simulink model "TxArray_2layers"  (R2021b)
settings: Solver=FixedStepDiscrete  StartTime=0.0  StopTime=100  FixedStep=1e-2  RelTol=1e-3  EnableMultiTasking=on
libraries: raspberrypiNetworklib x8, realtime_pacer_lib x1
settings Model: PacingRate=1000  Creator=Blade  LastModifiedBy=Blade
settings SolverCC: PositivePriorityOrder=on

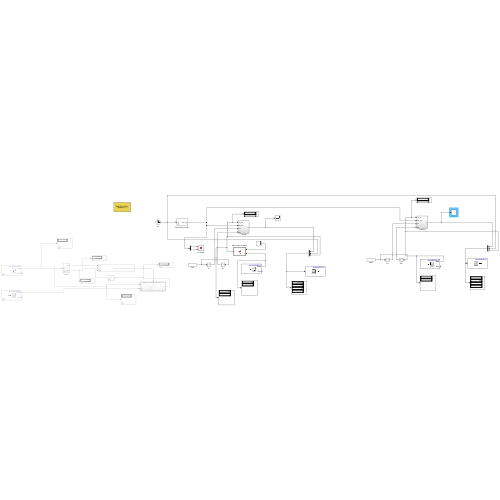
[thumbnail: Simulink's stored preview of the top-level diagram]
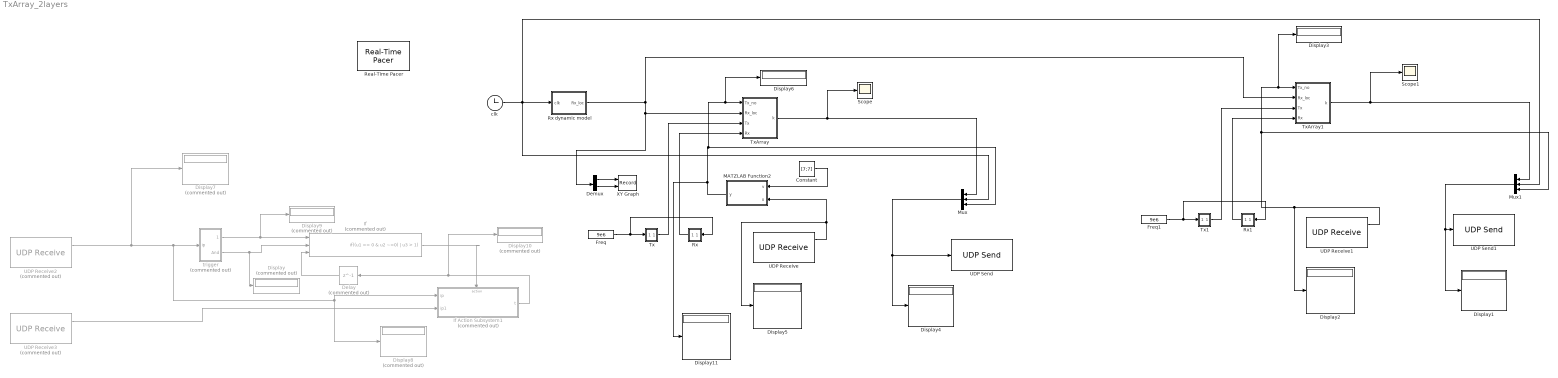
== system TxArray_2layers ==
  Constant : Constant  Value=[7;7]  VectorParams1D=off
  Delay : Delay  Commented=on  DelayLength=1  InitialCondition=0
  Demux : Demux  Outputs=2
  Display{,7..10} (5 alike) : Display  Commented=on
  Display{1..6,11} (7 alike) : Display
  Freq : Constant  Value=9e6
  Freq1 : Constant  Value=9e6
  If : If  Commented=on  NumInputs=3  IfExpression=(u1 == 0 & u2 ~=0) | u3 > 1  ShowElse=off
  If Action Subsystem1 : Subsystem  Commented=on  TreatAsAtomicUnit=on
  MATZLAB Function2 : MATLAB Function  TreatAsAtomicUnit=on
  Mux : Mux  Inputs=3
  Mux1 : Mux  Inputs=3
  Real-Time Pacer : realtime_pacer_lib/Real-Time Pacer  simTimePerRealTime=1
      settings: SourceProductName=Real-Time Pacer
  Rx : Subsystem  mask{dout=1/3*100e-3, phi=0.15, s=800e-6, w=1200e-6, CP=0, SR=0.01}
      mask prompts: dout "out diameter"; phi "fillfact"; s "track spacing"; w "track width"; CP "parasitic capacitance"; SR "source resistance"
      mask TypeOptions dout: Constant1/Value
      mask TypeOptions phi: Constant2/Value
      mask TypeOptions s: Constant3/Value
      mask TypeOptions w: Constant4/Value
      mask TypeOptions CP: Constant6/Value
      mask TypeOptions SR: Constant7/Value
  "Rx dynamic model " : Subsystem  mask{initx=1/2*100e-3*(7+1), inity=1/2*100e-3*(7+1), v_min=[0.01,0.01], v_max=[0.01,0.01]}
      mask prompts: initx "Rx initial x"; inity "Rx initial y"; v_min "Rx min speed"; v_max "Rx max speed"
      mask TypeOptions initx: Delay1/InitialCondition
      mask TypeOptions inity: Delay2/InitialCondition
      mask TypeOptions v_min: Constant/Value
      mask TypeOptions v_max: Constant1/Value
  Rx1 : Subsystem  mask{dout=1/3*100e-3, phi=0.15, s=800e-6, w=1200e-6, CP=0, SR=0.01}
      mask prompts: dout "out diameter"; phi "fillfact"; s "track spacing"; w "track width"; CP "parasitic capacitance"; SR "source resistance"
      mask TypeOptions dout: Constant1/Value
      mask TypeOptions phi: Constant2/Value
      mask TypeOptions s: Constant3/Value
      mask TypeOptions w: Constant4/Value
      mask TypeOptions CP: Constant6/Value
      mask TypeOptions SR: Constant7/Value
  Scope : Scope
  Scope1 : Scope
  Tx : Subsystem  mask{dout=100e-3, phi=0.25, s=3*2500e-6, w=2500e-6, CP=0, SR=0.01}
      mask prompts: dout "out diameter"; phi "fillfact"; s "track spacing"; w "track width"; CP "parasitic capacitance"; SR "source resistance"
      mask TypeOptions dout: Constant1/Value
      mask TypeOptions phi: Constant2/Value
      mask TypeOptions s: Constant3/Value
      mask TypeOptions w: Constant4/Value
      mask TypeOptions CP: Constant6/Value
      mask TypeOptions SR: Constant7/Value
  Tx1 : Subsystem  mask{dout=100e-3, phi=0.25, s=3*2500e-6, w=2500e-6, CP=0, SR=0.01}
      mask prompts: dout "out diameter"; phi "fillfact"; s "track spacing"; w "track width"; CP "parasitic capacitance"; SR "source resistance"
      mask TypeOptions dout: Constant1/Value
      mask TypeOptions phi: Constant2/Value
      mask TypeOptions s: Constant3/Value
      mask TypeOptions w: Constant4/Value
      mask TypeOptions CP: Constant6/Value
      mask TypeOptions SR: Constant7/Value
  TxArray : Subsystem
  TxArray1 : Subsystem
  UDP Receive : raspberrypiNetworklib/UDP Receive  localURL='0.0.0.0'  localPort=2000  remoteURL='0.0.0.0'  remotePort=-1  recvBufferSize=8192  signalDatatype=double  dims=2  isVarSize=off  showBlockingTime=off  blockingTime=0  sampletime=-1  blockPlatform=Raspberry Pi
      settings: SourceProductBaseCode=RASPPI
  UDP Receive1 : raspberrypiNetworklib/UDP Receive  localURL='0.0.0.0'  localPort=2100  remoteURL='0.0.0.0'  remotePort=-1  recvBufferSize=8192  signalDatatype=double  dims=2  isVarSize=off  showBlockingTime=off  blockingTime=0  sampletime=-1  blockPlatform=Raspberry Pi
      settings: SourceProductBaseCode=RASPPI
  UDP Receive2 : raspberrypiNetworklib/UDP Receive  Commented=on  localURL='0.0.0.0'  localPort=1000  remoteURL='0.0.0.0'  remotePort=-1  recvBufferSize=8192  signalDatatype=double  dims=4  isVarSize=off  showBlockingTime=off  blockingTime=0  sampletime=-1  blockPlatform=Raspberry Pi
      settings: SourceProductBaseCode=RASPPI
  UDP Receive3 : raspberrypiNetworklib/UDP Receive  Commented=on  localURL='0.0.0.0'  localPort=1100  remoteURL='0.0.0.0'  remotePort=-1  recvBufferSize=8192  signalDatatype=double  dims=4  isVarSize=off  showBlockingTime=off  blockingTime=0  sampletime=-1  blockPlatform=Raspberry Pi
      settings: SourceProductBaseCode=RASPPI
  UDP Send : raspberrypiNetworklib/UDP Send  remoteURL='172.20.10.3'  remotePort=1000  localURL='0.0.0.0'  localPortSource=Automatically determine  localPort=-1  sampletime=-1  blockPlatform=Raspberry Pi  separateLengthPort=0
      settings: SourceProductBaseCode=RASPPI
  UDP Send1 : raspberrypiNetworklib/UDP Send  remoteURL='172.20.10.3'  remotePort=1100  localURL='0.0.0.0'  localPortSource=Automatically determine  localPort=-1  sampletime=-1  blockPlatform=Raspberry Pi  separateLengthPort=0
      settings: SourceProductBaseCode=RASPPI
  XY Graph : Record  RecordToWorkspace=on  FileSettingsInternal="{\"entries\":[{\"content\":{\"excelSettings\":{\"content\":{},\"type\":\"Streamout.ExcelSettings\"}},\"type\":\"Streamout.FileSettingStorage\",\"uuid\":\"7534ccee-690c-42fe-b6df-7a669e2e1ce8\"}],\"packageUris\":[\"http://schema.mathworks.com/mf0/streamout_blocks/R2020a\"],\"version\":\"1.0\"}"  Layout=[1 1]  SignalsInternal="{\"entries\":[{\"content\":{\"signals\":[{\"content\":{\"blockPath\":[\"TxArray_2layers/XY Graph\"],\"channel\":[],\"dimensions\":[1],\"domain\":\"TxArray_2layers/XY Graph\",\"lineColor\":\"#a2142f\",\"plots\":[1],\"port\":1,\"sid\":[\"\"],\"signalID\":68672,\"signalName\":\"Demux:1\"},\"type\":\"RecordBlkView.Signal\",\"uuid\":\"5f268e60-035f-43e2-bfa9-f0f9b2fdeea8\"},{\"content\":{\"blockPath\":[\"TxArray_2layers/XY Graph\"],\"channel\":[],\"dimensions\":[1],\"domain\":\"TxArray_2layers/XY Graph\",\"lineColor\":\"#139fff\",\"plots\":[1],\"port\":2,\"sid\":[\"\"],\"signalID\":68676,\"signalName\":\"Demux:2\"},\"type\":\"RecordBlkView.Signal\",\"uuid\":\"7309d32f-aeee-4568-9c87-cfd759c20a08\"}]},\"type\":\"RecordBlkView.InputSignals\",\"uuid\":\"395885cf-4d5c-428c-bf2f-d29e5771728a\"}],\"packageUris\":[\"http://schema.mathworks.com/mf0/streamout_blocks/R2020a\"],\"version\":\"1.0\"}"  VisualizationBindings="{\"xyplotplugin\":{\"info\":[{\"series\":[{\"bindingParametersList\":[{\"parameter\":\"X-Axis\",\"signalID\":68672,\"signalName\":\"Demux:1\"},{\"parameter\":\"Y-Axis\",\"signalID\":68676,\"signalName\":\"Demux:2\"}],\"seriesID\":52649}],\"subplotID\":1}]}}"  CompatibilityTag=XY
  clk : Clock
  trigger : Subsystem  Commented=on
  wires:
  Mux1/1 -> Display1/1, UDP Send1/1
  Freq1/1 -> Rx1/1(In1), Tx1/1(In1)
  Rx1/1(Out1) -> TxArray1/4(Rx)
  UDP Receive/1 -> MATZLAB Function2/2(u), Display5/1
  Rx/1(Out1) -> TxArray/4(Rx)
  MATZLAB Function2/1(y) -> Display11/1, Mux/3, Display6/1, TxArray/1(Tx_no)
  Demux/2 -> XY Graph/2
  Tx/1(Out1) -> TxArray/3(Tx)
  Tx1/1(Out1) -> TxArray1/3(Tx)
  Freq/1 -> Rx/1(In1), Tx/1(In1)
  TxArray1/1(k) -> Scope1/1, Mux1/1
  Mux/1 -> Display4/1, UDP Send/1
  TxArray/1(k) -> Scope/1, Mux/1
  "Rx dynamic model "/1(Rx_loc) -> Demux/1, TxArray/2(Rx_loc), TxArray1/2(Rx_loc)
  clk/1 -> Mux1/2, Mux/2, "Rx dynamic model "/1(clk)
  Demux/1 -> XY Graph/1
  Constant/1 -> MATZLAB Function2/1(v)
  UDP Receive1/1 -> Mux1/3, Display3/1, TxArray1/1(Tx_no), Display2/1
  Delay/1 -> If/3
  trigger/1(mod) -> Display9/1, If/1
  If/1 -> If Action Subsystem1/Action
  trigger/2(And) -> Display/1, If/2
  If Action Subsystem1/1(t) -> Display10/1, Delay/1
  UDP Receive2/1 -> Display7/1, If Action Subsystem1/1(ip), Display8/1, trigger/1(ip)
  UDP Receive3/1 -> If Action Subsystem1/2(ip1)

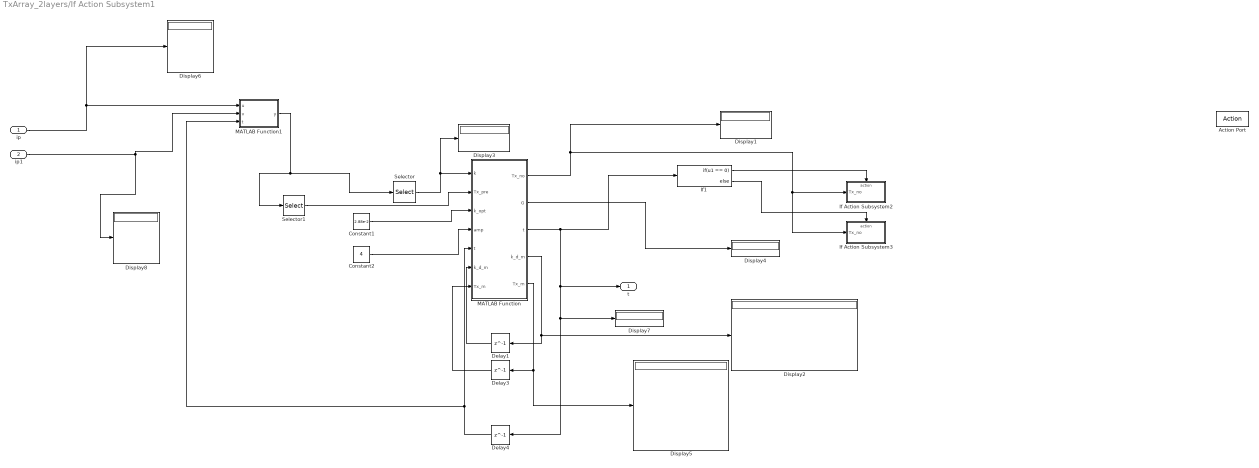
== system TxArray_2layers/If Action Subsystem1 ==
  ip : Inport
  ip1 : Inport  Port=2
  Action Port : ActionPort  ActionPortLabel=if((u1 == 0 & u2 ~=0) | u3 > 1)
  Constant1 : Constant  Value=2.88e-2
  Constant2 : Constant  Value=4
  Delay1 : Delay  DelayLength=1  InitialCondition=zeros(2,3)
  Delay3 : Delay  DelayLength=1  InitialCondition=zeros(8,2)
  Delay4 : Delay  DelayLength=1  InitialCondition=0
  Display{1..8} (8 alike) : Display
  If Action Subsystem2 : Subsystem  TreatAsAtomicUnit=on
  If Action Subsystem3 : Subsystem  TreatAsAtomicUnit=on
  If1 : If  IfExpression=u1 == 0
  MATLAB Function : MATLAB Function  TreatAsAtomicUnit=on
  MATLAB Function1 : MATLAB Function  TreatAsAtomicUnit=on
  Selector : Selector  InputPortWidth=4  IndexOptions=Index vector (dialog)  Indices=1  OutputSizes=1
  Selector1 : Selector  InputPortWidth=4  IndexOptions=Index vector (dialog)  Indices=[3;4]  OutputSizes=1
  t : Outport
  wires:
  MATLAB Function/5(Tx_m) -> Display5/1, Delay3/1
  MATLAB Function/2(G) -> Display4/1
  MATLAB Function/4(k_d_m) -> Delay1/1, Display2/1
  Delay1/1 -> MATLAB Function/6("k_d_m ")
  Selector/1 -> Display3/1, MATLAB Function/1(k)
  MATLAB Function/3(t) -> If1/1, Display7/1, Delay4/1, t/1
  Delay4/1 -> MATLAB Function1/3(t), MATLAB Function/5("t ")
  MATLAB Function/1(Tx_no) -> If Action Subsystem3/1(Tx_no), If Action Subsystem2/1(Tx_no), Display1/1
  Constant2/1 -> MATLAB Function/4(amp)
  Selector1/1 -> MATLAB Function/2(Tx_pre)
  Delay3/1 -> MATLAB Function/7("Tx_m ")
  MATLAB Function1/1(y) -> Selector1/1, Selector/1
  Constant1/1 -> MATLAB Function/3(k_opt)
  ip/1 -> MATLAB Function1/1(u), Display6/1
  If1/1 -> If Action Subsystem2/Action
  If1/2 -> If Action Subsystem3/Action
  ip1/1 -> Display8/1, MATLAB Function1/2(v)

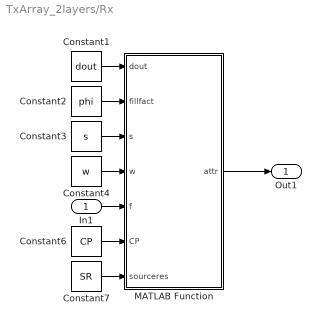
== system TxArray_2layers/Rx ==
  In1 : Inport
  Constant1 : Constant  Value=dout
  Constant2 : Constant  Value=phi
  Constant3 : Constant  Value=s
  Constant4 : Constant  Value=w
  Constant6 : Constant  Value=CP
  Constant7 : Constant  Value=SR
  MATLAB Function : MATLAB Function  TreatAsAtomicUnit=on
  Out1 : Outport
  wires:
  MATLAB Function/1(attr) -> Out1/1
  Constant7/1 -> MATLAB Function/7(sourceres)
  Constant1/1 -> MATLAB Function/1(dout)
  Constant2/1 -> MATLAB Function/2(fillfact)
  Constant3/1 -> MATLAB Function/3(s)
  Constant4/1 -> MATLAB Function/4(w)
  In1/1 -> MATLAB Function/5(f)
  Constant6/1 -> MATLAB Function/6(CP)

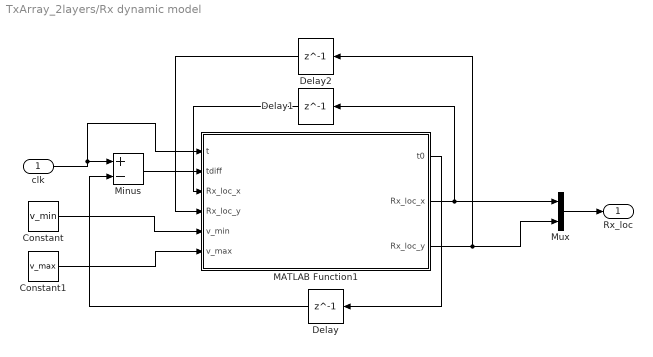
== system TxArray_2layers/Rx dynamic model  ==
  clk : Inport
  Constant : Constant  Value=v_min  VectorParams1D=off
  Constant1 : Constant  Value=v_max  VectorParams1D=off
  Delay : Delay  DelayLength=1  InitialCondition=0
  Delay1 : Delay  DelayLength=1  InitialCondition=initx
  Delay2 : Delay  DelayLength=1  InitialCondition=inity
  MATLAB Function1 : MATLAB Function  TreatAsAtomicUnit=on
  Minus : Sum  Inputs=+-
  Mux : Mux  Inputs=2
  Rx_loc : Outport
  wires:
  MATLAB Function1/3(Rx_loc_y) -> Delay2/1, Mux/2
  Delay/1 -> Minus/2
  clk/1 -> MATLAB Function1/1(t), Minus/1
  Delay2/1 -> MATLAB Function1/4("Rx_loc_y ")
  MATLAB Function1/1(t0) -> Delay/1
  Minus/1 -> MATLAB Function1/2(tdiff)
  Delay1/1 -> MATLAB Function1/3("Rx_loc_x ")
  MATLAB Function1/2(Rx_loc_x) -> Delay1/1, Mux/1
  Mux/1 -> Rx_loc/1
  Constant/1 -> MATLAB Function1/5(v_min)
  Constant1/1 -> MATLAB Function1/6(v_max)

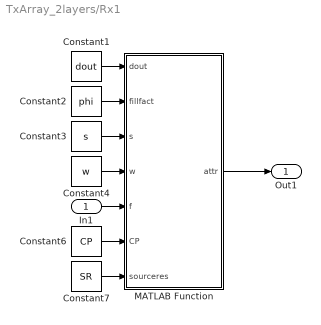
== system TxArray_2layers/Rx1 ==
  In1 : Inport
  Constant1 : Constant  Value=dout
  Constant2 : Constant  Value=phi
  Constant3 : Constant  Value=s
  Constant4 : Constant  Value=w
  Constant6 : Constant  Value=CP
  Constant7 : Constant  Value=SR
  MATLAB Function : MATLAB Function  TreatAsAtomicUnit=on
  Out1 : Outport
  wires:
  MATLAB Function/1(attr) -> Out1/1
  Constant7/1 -> MATLAB Function/7(sourceres)
  Constant1/1 -> MATLAB Function/1(dout)
  Constant2/1 -> MATLAB Function/2(fillfact)
  Constant3/1 -> MATLAB Function/3(s)
  Constant4/1 -> MATLAB Function/4(w)
  In1/1 -> MATLAB Function/5(f)
  Constant6/1 -> MATLAB Function/6(CP)

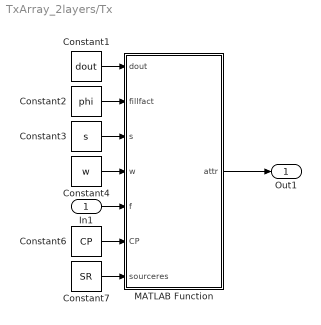
== system TxArray_2layers/Tx ==
  In1 : Inport
  Constant1 : Constant  Value=dout
  Constant2 : Constant  Value=phi
  Constant3 : Constant  Value=s
  Constant4 : Constant  Value=w
  Constant6 : Constant  Value=CP
  Constant7 : Constant  Value=SR
  MATLAB Function : MATLAB Function  TreatAsAtomicUnit=on
  Out1 : Outport
  wires:
  MATLAB Function/1(attr) -> Out1/1
  Constant7/1 -> MATLAB Function/7(sourceres)
  Constant1/1 -> MATLAB Function/1(dout)
  Constant2/1 -> MATLAB Function/2(fillfact)
  Constant3/1 -> MATLAB Function/3(s)
  Constant4/1 -> MATLAB Function/4(w)
  In1/1 -> MATLAB Function/5(f)
  Constant6/1 -> MATLAB Function/6(CP)

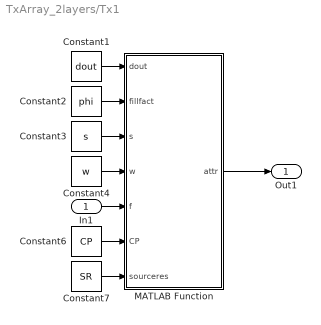
== system TxArray_2layers/Tx1 ==
  In1 : Inport
  Constant1 : Constant  Value=dout
  Constant2 : Constant  Value=phi
  Constant3 : Constant  Value=s
  Constant4 : Constant  Value=w
  Constant6 : Constant  Value=CP
  Constant7 : Constant  Value=SR
  MATLAB Function : MATLAB Function  TreatAsAtomicUnit=on
  Out1 : Outport
  wires:
  MATLAB Function/1(attr) -> Out1/1
  Constant7/1 -> MATLAB Function/7(sourceres)
  Constant1/1 -> MATLAB Function/1(dout)
  Constant2/1 -> MATLAB Function/2(fillfact)
  Constant3/1 -> MATLAB Function/3(s)
  Constant4/1 -> MATLAB Function/4(w)
  In1/1 -> MATLAB Function/5(f)
  Constant6/1 -> MATLAB Function/6(CP)

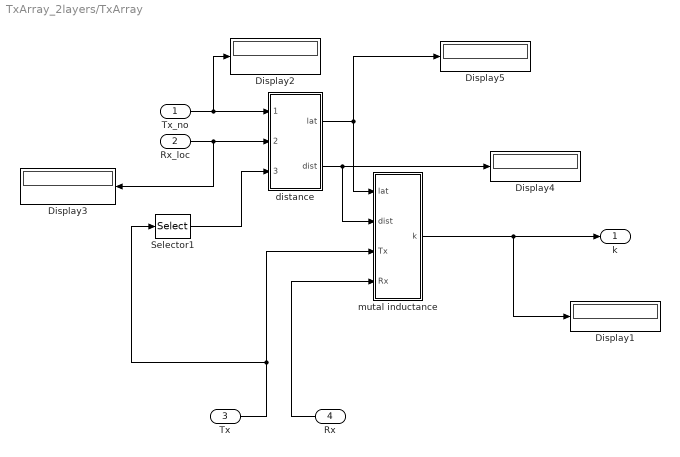
== system TxArray_2layers/TxArray ==
  Tx_no : Inport
  Rx_loc : Inport  Port=2
  Tx : Inport  Port=3
  Rx : Inport  Port=4
  " mutal inductance" : Subsystem
  Display{1..5} (5 alike) : Display
  Selector1 : Selector  InputPortWidth=14  IndexOptions=Index vector (dialog)  Indices=1  OutputSizes=1
  distance : Subsystem
  k : Outport
  wires:
  Tx/1 -> Selector1/1, " mutal inductance"/3(Tx)
  distance/1(lat) -> " mutal inductance"/1(lat), Display5/1
  Rx/1 -> " mutal inductance"/4(Rx)
  Tx_no/1 -> Display2/1, distance/1(Tx_no)
  Rx_loc/1 -> Display3/1, distance/2(Rx_loc)
  Selector1/1 -> distance/3(Tx_dia)
  " mutal inductance"/1(k) -> Display1/1, k/1
  distance/2(dist) -> " mutal inductance"/2(dist), Display4/1

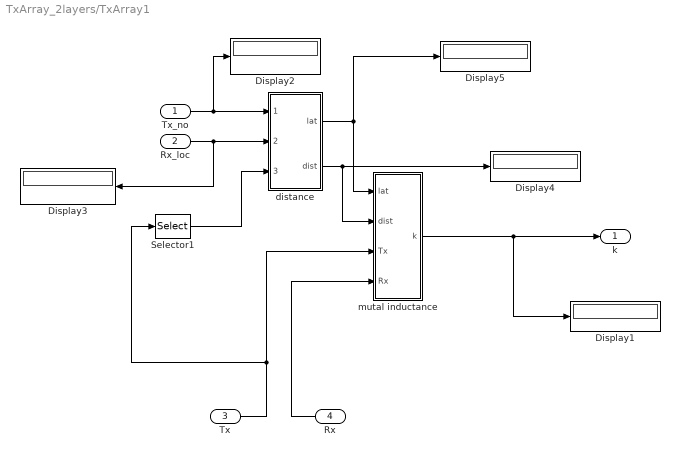
== system TxArray_2layers/TxArray1 ==
  Tx_no : Inport
  Rx_loc : Inport  Port=2
  Tx : Inport  Port=3
  Rx : Inport  Port=4
  " mutal inductance" : Subsystem
  Display{1..5} (5 alike) : Display
  Selector1 : Selector  InputPortWidth=14  IndexOptions=Index vector (dialog)  Indices=1  OutputSizes=1
  distance : Subsystem
  k : Outport
  wires:
  Tx/1 -> Selector1/1, " mutal inductance"/3(Tx)
  distance/1(lat) -> " mutal inductance"/1(lat), Display5/1
  Rx/1 -> " mutal inductance"/4(Rx)
  Tx_no/1 -> Display2/1, distance/1(Tx_no)
  Rx_loc/1 -> Display3/1, distance/2(Rx_loc)
  Selector1/1 -> distance/3(Tx_dia)
  " mutal inductance"/1(k) -> Display1/1, k/1
  distance/2(dist) -> " mutal inductance"/2(dist), Display4/1

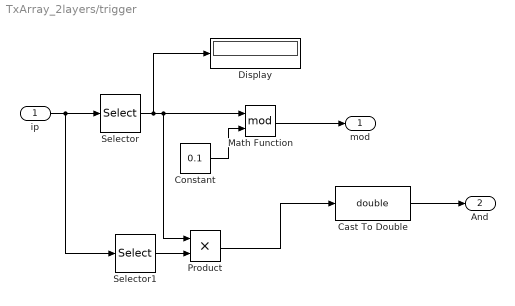
== system TxArray_2layers/trigger ==
  ip : Inport
  Cast To Double : DataTypeConversion  OutDataTypeStr=double
  Constant : Constant  Value=0.1
  Display : Display
  Math Function : Math  Operator=mod  SaturateOnIntegerOverflow=on
  Product : Product
  Selector : Selector  InputPortWidth=4  IndexOptions=Index vector (dialog)  Indices=2  OutputSizes=1
  Selector1 : Selector  InputPortWidth=4  IndexOptions=Index vector (dialog)  Indices=1  OutputSizes=1
  mod : Outport
  And : Outport  Port=2
  wires:
  Constant/1 -> Math Function/2
  Selector/1 -> Display/1, Product/1, Math Function/1
  ip/1 -> Selector1/1, Selector/1
  Math Function/1 -> mod/1
  Product/1 -> Cast To Double/1
  Selector1/1 -> Product/2
  Cast To Double/1 -> And/1

== system TxArray_2layers/If Action Subsystem1/If Action Subsystem2 ==
  Tx_no : Inport
  Action Port : ActionPort  ActionPortLabel=if(u1 == 0)
  UDP Send : raspberrypiNetworklib/UDP Send  remoteURL='172.20.10.2'  remotePort=2000  localURL='0.0.0.0'  localPortSource=Automatically determine  localPort=-1  sampletime=-1  blockPlatform=Raspberry Pi  separateLengthPort=0
      settings: SourceProductBaseCode=RASPPI
  wires:
  Tx_no/1 -> UDP Send/1

== system TxArray_2layers/If Action Subsystem1/If Action Subsystem3 ==
  Tx_no : Inport
  Action Port : ActionPort  ActionPortLabel=else
  UDP Send : raspberrypiNetworklib/UDP Send  remoteURL='172.20.10.2'  remotePort=2100  localURL='0.0.0.0'  localPortSource=Automatically determine  localPort=-1  sampletime=-1  blockPlatform=Raspberry Pi  separateLengthPort=0
      settings: SourceProductBaseCode=RASPPI
  wires:
  Tx_no/1 -> UDP Send/1

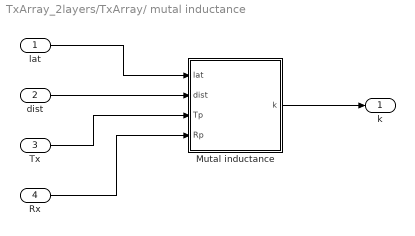
== system TxArray_2layers/TxArray/ mutal inductance ==
  lat : Inport
  dist : Inport  Port=2
  Tx : Inport  Port=3
  Rx : Inport  Port=4
  Mutal inductance : MATLAB Function  TreatAsAtomicUnit=on
  k : Outport
  wires:
  lat/1 -> Mutal inductance/1(lat)
  dist/1 -> Mutal inductance/2(dist)
  Tx/1 -> Mutal inductance/3(Tp)
  Rx/1 -> Mutal inductance/4(Rp)
  Mutal inductance/1(k) -> k/1

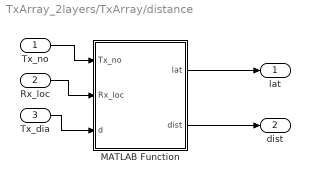
== system TxArray_2layers/TxArray/distance ==
  Tx_no : Inport
  Rx_loc : Inport  Port=2
  Tx_dia : Inport  Port=3
  MATLAB Function : MATLAB Function  TreatAsAtomicUnit=on
  lat : Outport
  dist : Outport  Port=2
  wires:
  Tx_dia/1 -> MATLAB Function/3(d)
  Tx_no/1 -> MATLAB Function/1(Tx_no)
  Rx_loc/1 -> MATLAB Function/2(Rx_loc)
  MATLAB Function/1(lat) -> lat/1
  MATLAB Function/2(dist) -> dist/1

== system TxArray_2layers/TxArray1/ mutal inductance ==
  lat : Inport
  dist : Inport  Port=2
  Tx : Inport  Port=3
  Rx : Inport  Port=4
  Mutal inductance : MATLAB Function  TreatAsAtomicUnit=on
  k : Outport
  wires:
  lat/1 -> Mutal inductance/1(lat)
  dist/1 -> Mutal inductance/2(dist)
  Tx/1 -> Mutal inductance/3(Tp)
  Rx/1 -> Mutal inductance/4(Rp)
  Mutal inductance/1(k) -> k/1

== system TxArray_2layers/TxArray1/distance ==
  Tx_no : Inport
  Rx_loc : Inport  Port=2
  Tx_dia : Inport  Port=3
  MATLAB Function : MATLAB Function  TreatAsAtomicUnit=on
  lat : Outport
  dist : Outport  Port=2
  wires:
  Tx_dia/1 -> MATLAB Function/3(d)
  Tx_no/1 -> MATLAB Function/1(Tx_no)
  Rx_loc/1 -> MATLAB Function/2(Rx_loc)
  MATLAB Function/1(lat) -> lat/1
  MATLAB Function/2(dist) -> dist/1

== matlab function TxArray_2layers/TxArray/distance/MATLAB Function ==
  data: Tx_no input; Rx_loc input; d input; lat output; dist output
function [lat, dist] = distance(Tx_no, Rx_loc, d)

coder.extrinsic('lat_dist');
coder.extrinsic('vertical_dist');


lat = 0;
dist = 0;

lat = lat_dist(Tx_no, Rx_loc,d);
dist = vertical_dist(Tx_no);
dist = dist + 5e-2;
end

== matlab function TxArray_2layers/If Action Subsystem1/MATLAB Function1 ==
  data: u input; y output; v input; t input
function y = fcn(u,v,t)
if t<=2
    y = u;
else
    y = v;
end

== matlab function TxArray_2layers/If Action Subsystem1/MATLAB Function ==
  data: k input; Tx_pre input; Tx_no output; G output; t output; k_opt input; amp input; t input; k_d_m output; k_d_m input; Tx_m input; Tx_m output
function [Tx_no,G,t,k_d_m,Tx_m] = Controller(k,Tx_pre,k_opt,amp,t,k_d_m,Tx_m)

k_diff = abs(k_opt-k)/k_opt;
Tx_pre = Tx_pre';

if t == 0
   

    t = t+1;
    k_d_m(1,:)  = [k_diff,Tx_pre];
    k_d_m(2,:)  = [k_diff,Tx_pre];

    
else

    if k_diff < k_d_m(2,1)

       k_d_m(2,:)  = [k_diff,Tx_pre];

    end

end

G = round(amp*k_d_m(1,1));  
Tx_fix = k_d_m(1,2:3)';

if t < 10
    
    if t < 9

        if G ==0
            Tx_no = [0;0];
        else

            dir_att = [-1,-1; -1,0; 0,-1; 1,1; 1,0; 0,1; 1,-1; -1,1];
            
            
            Tx_no =G*dir_att(t,:)'+Tx_fix;
        
            Tx_m (t,:) = Tx_no;
        end

    else

         Tx_no = [0;0]; % off

    end

    t =t+1;

else
    
    
    Tx_no = k_d_m(2,2:3)';

    t =0;
   
 
end

== matlab function TxArray_2layers/Rx1/MATLAB Function ==
  data: dout input; attr output; fillfact input; s input; w input; f input; CP input; sourceres input
function attr = PCBPhySim(dout,fillfact,s,w,f,CP,sourceres)


y = PCBCoil(dout,fillfact,s,w,f,CP,'square',sourceres);

attr = [y.dout,
    y.din,
    y.fillfact,
    y.w,
    y.s,
    y.n,
    y.L,
    y.Rs,
    y.Q,
    y.C,
    y.CP,
    y.coilZ,
    y.fSRF
    y.f];

== matlab function TxArray_2layers/Tx1/MATLAB Function ==
  data: dout input; attr output; fillfact input; s input; w input; f input; CP input; sourceres input
function attr = PCBPhySim(dout,fillfact,s,w,f,CP,sourceres)


y = PCBCoil(dout,fillfact,s,w,f,CP,'square',sourceres);

attr = [y.dout,
    y.din,
    y.fillfact,
    y.w,
    y.s,
    y.n,
    y.L,
    y.Rs,
    y.Q,
    y.C,
    y.CP,
    y.coilZ,
    y.fSRF
    y.f];

== matlab function TxArray_2layers/TxArray1/ mutal inductance/Mutal inductance ==
  data: lat input; dist input; Tp input; Rp input; k output
function  k = solenoid_MI(lat,dist,Tp,Rp)


coder.extrinsic('MI');

% M = 0;
k = 0;

[~,k] = MI(lat,dist,Tp,Rp);

if k < 0
    k = 0;
end

end

== matlab function TxArray_2layers/TxArray1/distance/MATLAB Function ==
  data: Tx_no input; Rx_loc input; d input; lat output; dist output
function [lat, dist] = distance(Tx_no, Rx_loc, d)

coder.extrinsic('lat_dist');
coder.extrinsic('vertical_dist');


lat = 0;
dist = 0;

lat = lat_dist(Tx_no, Rx_loc,d);
dist = vertical_dist(Tx_no);
dist = dist + 5e-2;
end

== matlab function TxArray_2layers/TxArray/ mutal inductance/Mutal inductance ==
  data: lat input; dist input; Tp input; Rp input; k output
function  k = solenoid_MI(lat,dist,Tp,Rp)


coder.extrinsic('MI');

% M = 0;
k = 0;

[~,k] = MI(lat,dist,Tp,Rp);

if k < 0
    k = 0;
end

end

== matlab function TxArray_2layers/Tx/MATLAB Function ==
  data: dout input; attr output; fillfact input; s input; w input; f input; CP input; sourceres input
function attr = PCBPhySim(dout,fillfact,s,w,f,CP,sourceres)


y = PCBCoil(dout,fillfact,s,w,f,CP,'square',sourceres);

attr = [y.dout,
    y.din,
    y.fillfact,
    y.w,
    y.s,
    y.n,
    y.L,
    y.Rs,
    y.Q,
    y.C,
    y.CP,
    y.coilZ,
    y.fSRF
    y.f];

== matlab function TxArray_2layers/MATZLAB Function2 ==
  data: v input; u input; y output
function y = fcn(v, u)
if u==0

    y = v;
else 
    y = u;
end

== matlab function TxArray_2layers/Rx/MATLAB Function ==
  data: dout input; attr output; fillfact input; s input; w input; f input; CP input; sourceres input
function attr = PCBPhySim(dout,fillfact,s,w,f,CP,sourceres)


y = PCBCoil(dout,fillfact,s,w,f,CP,'square',sourceres);

attr = [y.dout,
    y.din,
    y.fillfact,
    y.w,
    y.s,
    y.n,
    y.L,
    y.Rs,
    y.Q,
    y.C,
    y.CP,
    y.coilZ,
    y.fSRF
    y.f];

== matlab function TxArray_2layers/Rx dynamic model /MATLAB Function1 ==
  data: t input; tdiff input; t0 output; Rx_loc_x output; Rx_loc_x input; Rx_loc_y input; Rx_loc_y output; v_min input; v_max input
function [t0, Rx_loc_x, Rx_loc_y] = dynamic_on_TxArray(t, tdiff, Rx_loc_x, Rx_loc_y, v_min, v_max)
% if t>=0 && t < 8
%     tdiff = 0;
% elseif t>=10 && t < 19
%     tdiff = 0;
% elseif t>=20 && t < 29
%     tdiff = 0;
% elseif t>=30 && t < 39
%     tdiff = 0;   
% elseif t>=40 && t < 49
%     tdiff = 0;
% elseif t>=50 && t < 59
%     tdiff = 0;
% elseif t>=60 && t < 69
%     tdiff = 0;
% elseif t>=70 && t < 79
%     tdiff = 0;
% elseif t>=80 && t < 89
%     tdiff = 0;
% elseif t>=90 && t < 99
%     tdiff = 0;
% end

d = 0;
Rx_loc = [Rx_loc_x,Rx_loc_y];
coder.extrinsic('dynamic');
Rx_loc = dynamic(tdiff,Rx_loc,v_min,v_max);
Rx_loc_x = 0;
Rx_loc_y = 0;
Rx_loc_x = Rx_loc(1);
Rx_loc_y = Rx_loc(2);

t0 = t;
